simulink model "CRC6BitCheckSum"  (Simulink 8.3)
settings: Solver=ode45  StartTime=0.0  StopTime=10.0  RelTol=1e-3
libraries: simulink x4
settings Model: Creator=ohc  LastModifiedBy=ohc
settings DataIOCC: SignalLoggingSaveFormat=Dataset
settings DebuggingCC: UnderspecifiedInitializationDetection=Simplified  StateNameClashWarn=none
settings GRTTargetCC: CombineOutputUpdateFcns=on  GRTInterface=off

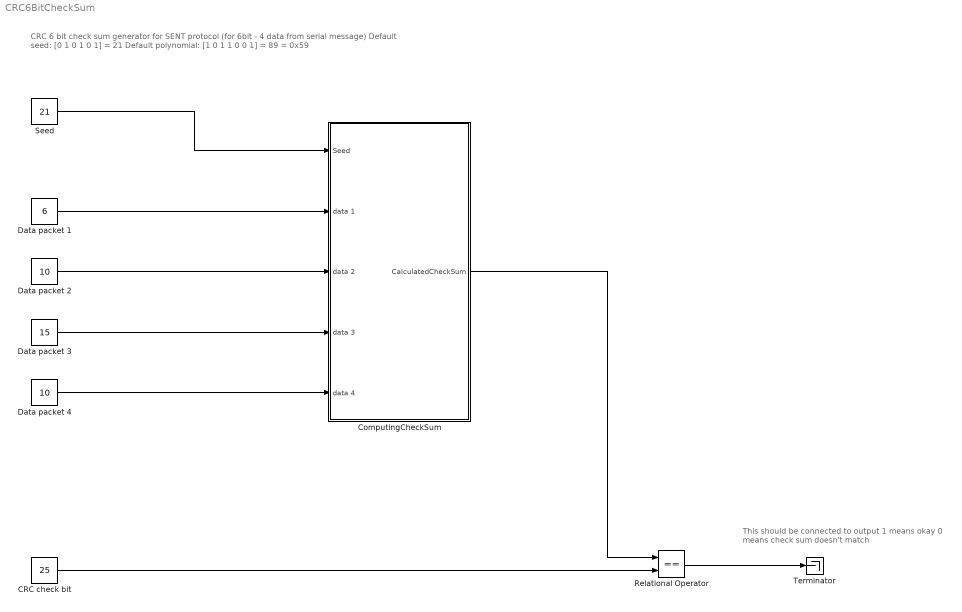
== system CRC6BitCheckSum ==
  note: This should be connected to output
      | 1 means okay 0 means check sum doesn't match
  note: CRC 6 bit check sum generator for SENT protocol (for 6bit - 4 data from serial message)
      | Default seed:  [0 1 0 1 0 1] = 21
      | Default polynomial: [1 0 1 1 0 0 1] =  89 = 0x59
  CRC check bit : Constant  Value=25  OutMin=0  OutMax=63  OutDataTypeStr=uint8
  ComputingCheckSum : Subsystem
  Data packet 1 : Constant  Value=6  OutMin=0  OutMax=63  OutDataTypeStr=uint8
  Data packet 2 : Constant  Value=10  OutMin=0  OutMax=63  OutDataTypeStr=uint8
  Data packet 3 : Constant  Value=15  OutMin=0  OutMax=63  OutDataTypeStr=uint8
  Data packet 4 : Constant  Value=10  OutMin=0  OutMax=63  OutDataTypeStr=uint8
  Relational Operator : RelationalOperator  Operator===  OutDataTypeStr=boolean
  Seed : Constant  Value=21  OutMin=0  OutMax=63  OutDataTypeStr=uint8
  Terminator : Terminator
  wires:
  Seed/1 -> ComputingCheckSum/1(Seed)
  Data packet 1/1 -> ComputingCheckSum/2(data 1)
  Data packet 2/1 -> ComputingCheckSum/3(data 2)
  Data packet 3/1 -> ComputingCheckSum/4(data 3)
  Data packet 4/1 -> ComputingCheckSum/5(data 4)
  CRC check bit/1 -> Relational Operator/2
  ComputingCheckSum/1(CalculatedCheckSum) -> Relational Operator/1
  Relational Operator/1 -> Terminator/1

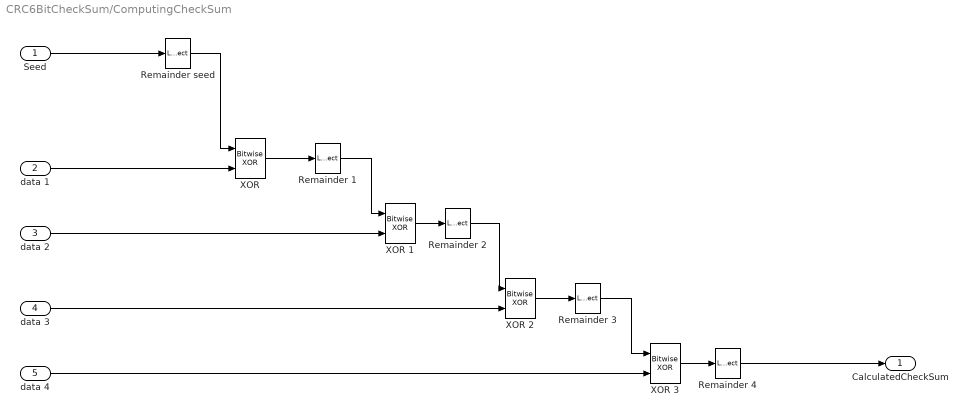
== system CRC6BitCheckSum/ComputingCheckSum ==
  Seed : Inport
  data 1 : Inport  Port=2
  data 2 : Inport  Port=3
  data 3 : Inport  Port=4
  data 4 : Inport  Port=5
  Remainder {1..4} (4 alike) : LookupNDDirect  NumberOfTableDimensions=1  Table="[0\t25\t50\t43\t61\t36\t15\t22\t35\t58\t17\t8\t30\t7\t44\t53\t31\t6\t45\t52\t34\t59\t16\t9\t60\t37\t14\t23\t1\t24\t51\t42\t62\t39\t12\t21\t3\t26\t49\t40\t29\t4\t47\t54\t32\t57\t18\t11\t33\t56\t19\t10\t28\t5\t46\t55\t2\t27\t48\t41\t63\t38\t13\t20]"  TableMin=0  TableMax=63  TableDataTypeStr=uint8
  Remainder seed : LookupNDDirect  NumberOfTableDimensions=1  Table="[0\t25\t50\t43\t61\t36\t15\t22\t35\t58\t17\t8\t30\t7\t44\t53\t31\t6\t45\t52\t34\t59\t16\t9\t60\t37\t14\t23\t1\t24\t51\t42\t62\t39\t12\t21\t3\t26\t49\t40\t29\t4\t47\t54\t32\t57\t18\t11\t33\t56\t19\t10\t28\t5\t46\t55\t2\t27\t48\t41\t63\t38\t13\t20]"  TableMin=0  TableMax=63  TableDataTypeStr=uint8
  XOR {,1..3} (4 alike) : simulink/Logic and Bit Operations/Bitwise Operator  logicop=XOR  UseBitMask=off  NumInputPorts=2  BitMask=bin2dec('11011001')  BitMaskRealWorld=Stored Integer
  CalculatedCheckSum : Outport
  wires:
  data 3/1 -> XOR 2/2
  XOR 1/1 -> Remainder 2/1
  data 1/1 -> "XOR "/2
  Seed/1 -> Remainder seed/1
  Remainder seed/1 -> "XOR "/1
  Remainder 2/1 -> XOR 2/1
  data 4/1 -> XOR 3/2
  XOR 2/1 -> Remainder 3/1
  Remainder 1/1 -> XOR 1/1
  XOR 3/1 -> Remainder 4/1
  data 2/1 -> XOR 1/2
  Remainder 3/1 -> XOR 3/1
  "XOR "/1 -> Remainder 1/1
  Remainder 4/1 -> CalculatedCheckSum/1
